simulink model "naibaoOSTBC_42"  (R2018a)
settings: Solver=VariableStepAuto  StartTime=0.0  StopTime=1  RelTol=1e-3
model workspace (MAT data in the model file):
  FrameLen = 80
  SampleTime = 0.001
  maxNumBits = 100000000
  maxNumErrs = 1000
libraries: commdigbbndpm3 x2, commmimo x2, commchan3 x1, commrandsrc3 x1, commsink2 x1
settings Model: Creator=myste  LastModifiedBy=myste

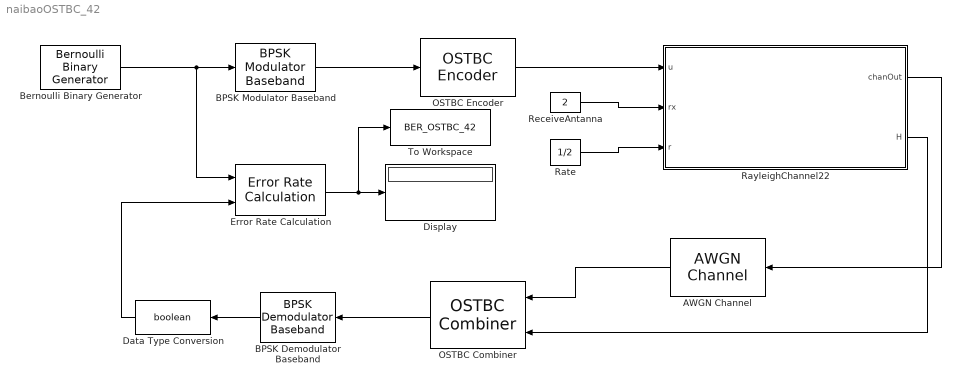
== system naibaoOSTBC_42 ==
  AWGN Channel : commchan3/AWGN Channel  InputProcessing=Columns as channels (frame based)  seed=67  noiseMode="Signal to noise ratio  (Eb/No)"  EbNodB=EbNo  EsNodB=10  SNRdB=10  bitsPerSym=1  Ps=1  Tsym=SampleTime  variance=1
  BPSK Demodulator Baseband : commdigbbndpm3/BPSK Demodulator Baseband  DecType=Hard decision  VarSource=Dialog  Variance=1  Ph=0  outDtype=Inherit via internal rule  derotateFactorWordLen=16  derotateFactorDataTypeStr=Inherit: Same word length as input  derotateFactorLastDataTypeStr=Inherit: Same word length as input
  BPSK Modulator Baseband : commdigbbndpm3/BPSK Modulator Baseband  Ph=0  outDtype=double  outWordLen=16  outUDDataType=sfix(16)  outFracLenMode=Best precision  outFracLen=15  outDataTypeStr=double  outLastDataTypeStr=double
  Bernoulli Binary Generator : commrandsrc3/Bernoulli Binary Generator  ProbabilityOfZero=0.5  SeedSource=Auto  Seed=0  SampleTime=SampleTime  SamplesPerFrame=FrameLen  OutputDataType=boolean  SimulateUsing=Interpreted execution
  Data Type Conversion : DataTypeConversion  OutDataTypeStr=boolean
  Display : Display
  Error Rate Calculation : commsink2/Error Rate Calculation  N=0  st_delay=0  cp_mode=Entire frame  subframe=[]  PMode=Port  WsName=ErrorVec  RsMode2=off  stop=on  numErr=maxNumErrs  maxBits=maxNumBits
  OSTBC Combiner : commmimo/OSTBC Combiner  numTx=4  rate=1/2  numRx=2  roundingMode=Floor  overflowMode=Wrap  OvFlMode=off  OvFlModeLastStrValue=off  crossProductWordLen=32  crossProductFracLen=16  crossSumWordLen=32  crossSumFracLen=16  egyProductWordLen=32  egyProductFracLen=16  egySumWordLen=32  egySumFracLen=16  divisionWordLen=32  divisionFracLen=16  divisionDataTypeStr=Inherit: Same as accumulator  divisionLastDataTypeStr=Inherit: Same as accumulator
      settings: SourceProductName=Communications System Toolbox  SourceProductBaseCode=CM
  OSTBC Encoder : commmimo/OSTBC Encoder  numTx=4  rate=1/2  overflowMode=Wrap  OvFlMode=off  OvFlModeLastStrValue=off
      settings: SourceProductName=Communications System Toolbox  SourceProductBaseCode=CM
  Rate : Constant  Value=1/2
  RayleighChannel22 : MATLAB Function  TreatAsAtomicUnit=on
  ReceiveAntanna : Constant  Value=2
  To Workspace : ToWorkspace  VariableName=BER_OSTBC_42  SampleTime=-1
      settings: MaxDataPoints=1  Save2DSignal=2-D array (concatenate along first dimension)
  wires:
  Bernoulli Binary Generator/1 -> Error Rate Calculation/1, BPSK Modulator Baseband/1
  BPSK Modulator Baseband/1 -> OSTBC Encoder/1
  OSTBC Encoder/1 -> RayleighChannel22/1(u)
  ReceiveAntanna/1 -> RayleighChannel22/2(rx)
  RayleighChannel22/2(H) -> OSTBC Combiner/2
  OSTBC Combiner/1 -> BPSK Demodulator Baseband/1
  RayleighChannel22/1(chanOut) -> AWGN Channel/1
  AWGN Channel/1 -> OSTBC Combiner/1
  Error Rate Calculation/1 -> To Workspace/1, Display/1
  BPSK Demodulator Baseband/1 -> Data Type Conversion/1
  Data Type Conversion/1 -> Error Rate Calculation/2
  Rate/1 -> RayleighChannel22/3(r)

== matlab function naibaoOSTBC_42/RayleighChannel22 ==
  data: u input; chanOut output; H output; rx input; r input
function [chanOut,H] = RayleighChannel22(u,rx,r)
%得到Rayleigh信道，u为发射天线的信息，rx为接收天线的个数,r为编码速率
%% 初始化参数
% 获取输入帧长,输入天线数
s=size(u);
FrameLength=s(1);
N=s(2);
%接收天线数
M=rx;
%两个时隙中信道参数保持不变
Num=0;
%生成信道矩阵
H = complex( zeros(FrameLength, N, 2) );
%% 生成信道并计算输出
%计算Num
if s(2)==2 
    Num=4;
end
if s(2)==4 && r==3/4
    Num=8;
end
if s(2)==4 && r==1/2
    Num=16;
end
%生成分组中，第一个分组中的信道增益
H(1:Num:end, :, :) = (randn(FrameLength/Num, N, M) + ...
                         1i*randn(FrameLength/Num, N, M))/sqrt(2);
%assume held constant for other symbol periods
for i=2:Num
    H(i:Num:end, :, :) = H(1:Num:end, :, :);
end
%第一个接收天线的信道矩阵
H21 = H(:,:,1)/sqrt(2);
%第二个接收天线的信道矩阵
H22 = H(:,:,2)/sqrt(2);
%输出接收天线1信号
chanOut21 = sum(H21.* u, 2);
%输出接收天线2信号
chanOut22 = sum(H22.* u, 2);
%输出信号
chanOut=[chanOut21,chanOut22];
